simulink model "BioTac_SlipDetection_Simplified"  (R2025b)
settings: Solver=FixedStepDiscrete  StartTime=0.0  StopTime=SIM_DURATION  FixedStep=0.001  RelTol=1e-3
settings Model: PacingRate=0.200000  Creator=gawin  LastModifiedBy=gawin

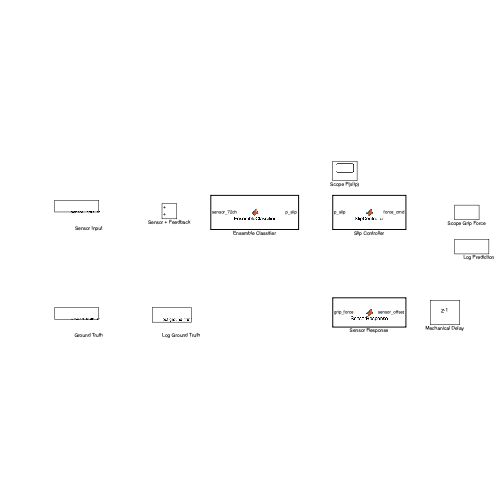
[thumbnail: Simulink's stored preview of the top-level diagram]
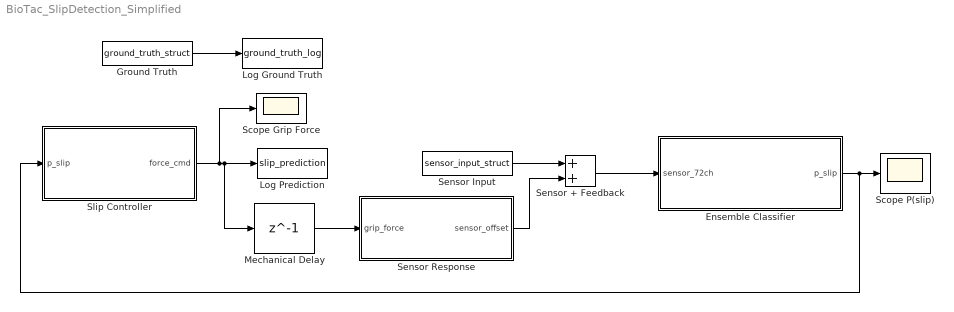
== system BioTac_SlipDetection_Simplified ==
  Ensemble Classifier : MATLAB Function  TreatAsAtomicUnit=on
  Ground Truth : FromWorkspace  VariableName=ground_truth_struct  SampleTime=0.001  Interpolate=off  OutputAfterFinalValue=Cyclic repetition
  Log Ground Truth : ToWorkspace  VariableName=ground_truth_log  SaveFormat=Timeseries  SampleTime=-1
  Log Prediction : ToWorkspace  VariableName=slip_prediction  SaveFormat=Timeseries  SampleTime=-1
  Mechanical Delay : Delay  DelayLength=1  InitialCondition=3.0
  Scope Grip Force : Scope
  Scope P(slip) : Scope
  Sensor + Feedback : Sum
  Sensor Input : FromWorkspace  VariableName=sensor_input_struct  SampleTime=0.001  Interpolate=off  OutputAfterFinalValue=Cyclic repetition
  Sensor Response : MATLAB Function  TreatAsAtomicUnit=on
  Slip Controller : MATLAB Function  TreatAsAtomicUnit=on
  wires:
  Ensemble Classifier/1(p_slip) -> Scope P(slip)/1, Slip Controller/1(p_slip)
  Sensor Response/1(sensor_offset) -> Sensor + Feedback/2
  Sensor Input/1 -> Sensor + Feedback/1
  Mechanical Delay/1 -> Sensor Response/1(grip_force)
  Sensor + Feedback/1 -> Ensemble Classifier/1(sensor_72ch)
  Slip Controller/1(force_cmd) -> Mechanical Delay/1, Log Prediction/1, Scope Grip Force/1
  Ground Truth/1 -> Log Ground Truth/1

== matlab function BioTac_SlipDetection_Simplified/Ensemble Classifier ==
  data: sensor_72ch input; p_slip output
function p_slip = EnsembleClassifier(sensor_72ch)
%#codegen
coder.extrinsic('predict'); coder.extrinsic('load_finger_net');
p_slip = 0; scores1 = zeros(1, 2); scores2 = zeros(1, 2); scores3 = zeros(1, 2);
persistent net1 net2 net3
if isempty(net1)
    net1 = load_finger_net(1); net2 = load_finger_net(2); net3 = load_finger_net(3);
end
if numel(sensor_72ch) == 72
    x = double(sensor_72ch(:)');
    scores1 = double(predict(net1, x(1:24))); scores2 = double(predict(net2, x(25:48))); scores3 = double(predict(net3, x(49:72)));
    p_slip = (scores1(2) + scores2(2) + scores3(2)) / 3;
end; end

== matlab function BioTac_SlipDetection_Simplified/Sensor Response ==
  data: grip_force input; sensor_offset output
function sensor_offset = SensorResponse(grip_force)
%#codegen
sensor_offset = zeros(1, 72);
f_norm = max(0, min(1, (grip_force - 3.0) / 5.0));

% INCREASED FEEDBACK: -2.0 shift completely suppresses the AI slip prediction
sensor_offset = (-2.0 * f_norm) * ones(1, 72);
end

== matlab function BioTac_SlipDetection_Simplified/Slip Controller ==
  data: p_slip input; force_cmd output
function force_cmd = SlipController(p_slip)
%#codegen
persistent hold_timer
if isempty(hold_timer), hold_timer = 0; end

% Config: 50ms hold (50 samples), 0.5 threshold
if p_slip > 0.5
    hold_timer = 50;
end

% Output logic: 8N if timer active, 3N otherwise
if hold_timer > 0
    force_cmd = 8.0;
    hold_timer = hold_timer - 1;
else
    force_cmd = 3.0;
end; end
